simulink library "CTRL_SPECCTRL_FB_STRAT1_REG"  (R2024b)
settings: Solver=VariableStepAuto  StartTime=0.0  StopTime=10.0  RelTol=1e-3
undefined symbols (not defined in the file or in its folder): CTRL_SPECCTRL_FB_STRAT1_REG_DmpLoLim_p100, CTRL_SPECCTRL_FB_STRAT1_REG_DmpUpLim_p100
libraries: slpidlib x4, simulink x4
settings Model: Creator=blatak  LastModifiedBy=blatak

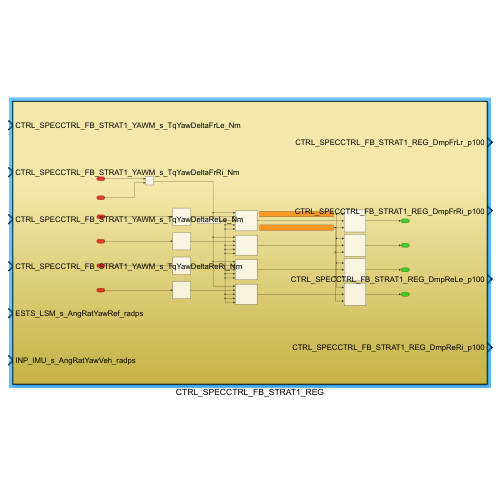
[thumbnail: Simulink's stored preview of the top-level diagram]
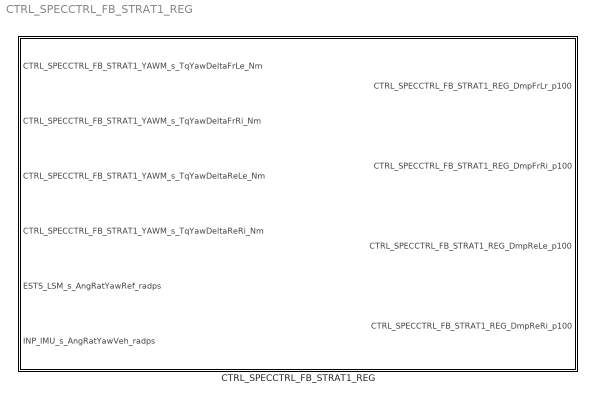
== system CTRL_SPECCTRL_FB_STRAT1_REG ==
  CTRL_SPECCTRL_FB_STRAT1_REG : Subsystem

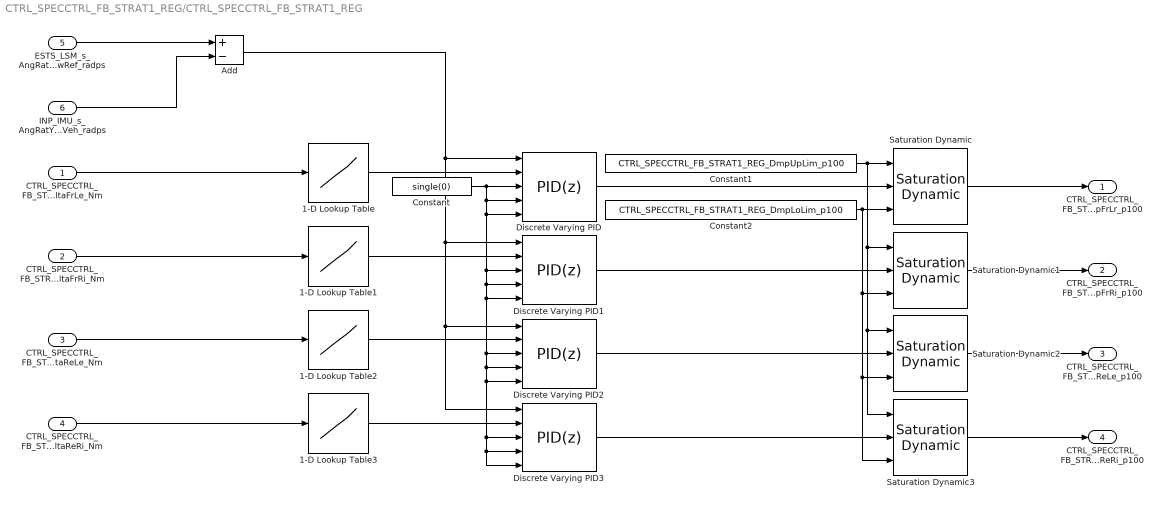
== system CTRL_SPECCTRL_FB_STRAT1_REG/CTRL_SPECCTRL_FB_STRAT1_REG ==
  CTRL_SPECCTRL_FB_STRAT1_YAWM_s_TqYawDeltaFrLe_Nm : Inport
  CTRL_SPECCTRL_FB_STRAT1_YAWM_s_TqYawDeltaFrRi_Nm : Inport  Port=2
  CTRL_SPECCTRL_FB_STRAT1_YAWM_s_TqYawDeltaReLe_Nm : Inport  Port=3
  CTRL_SPECCTRL_FB_STRAT1_YAWM_s_TqYawDeltaReRi_Nm : Inport  Port=4
  ESTS_LSM_s_AngRatYawRef_radps : Inport  Port=5
  INP_IMU_s_AngRatYawVeh_radps : Inport  Port=6
  1-D Lookup Table{,1..3} (4 alike) : Lookup_n-D  NumberOfTableDimensions=1  BreakpointsForDimension1=[-5:5]  Table=tanh([-5:5])  InternalRulePriority=Speed  RndMeth=Simplest
  Add : Sum  Inputs=+-
  Constant : Constant  Value=single(0)
  Constant1 : Constant  Value=CTRL_SPECCTRL_FB_STRAT1_REG_DmpUpLim_p100
  Constant2 : Constant  Value=CTRL_SPECCTRL_FB_STRAT1_REG_DmpLoLim_p100
  Discrete Varying PID{,1..3} (4 alike) : slpidlib/PID Controller  Controller=PID  Form=Parallel  TimeDomain=Discrete-time  UseExternalTs=off  SampleTime=-1  IntegratorMethod=Forward Euler  FilterMethod=Forward Euler  ControllerParametersSource=external  P=1  I=1  UseKiTs=off  D=0  UseExternalDerivativeSource=off  N=100  UseFilter=on  TunerSelectOption=Transfer Function Based (PID Tuner App)  InitialConditionSource=internal  InitialConditionForIntegrator=0  InitialConditionForFilter=0  DifferentiatorICPrevScaledInput=0  ExternalReset=none  TrackingMode=off  Kt=1  LimitOutput=off  SatLimitsSource=internal  UpperSaturationLimit=inf  LowerSaturationLimit=-inf  LinearizeAsGain=on  AntiWindupMode=none  Kb=1  LimitIntegrator=off  UpperIntegratorSaturationLimit=inf  LowerIntegratorSaturationLimit=-inf  POutMin=[]  POutMax=[]  IOutMin=[]  IOutMax=[]  DOutMin=[]  DOutMax=[]  NOutMin=[]  NOutMax=[]  SumOutMin=[]  SumOutMax=[]  SaturationOutMin=[]  SaturationOutMax=[]  PParamMin=[]  PParamMax=[]  IParamMin=[]  IParamMax=[]  DParamMin=[]  DParamMax=[]  NParamMin=[]  NParamMax=[]  KbParamMin=[]  KbParamMax=[]  KtParamMin=[]  KtParamMax=[]  KbOutMin=[]  KbOutMax=[]  KtOutMin=[]  KtOutMax=[]  IntegratorOutMin=[]  IntegratorOutMax=[]  FilterOutMin=[]  FilterOutMax=[]  SumI1OutMin=[]  SumI1OutMax=[]  SumI2OutMin=[]  SumI2OutMax=[]  SumI3OutMin=[]  SumI3OutMax=[]  SumI4OutMin=[]  SumI4OutMax=[]  SumDOutMin=[]  SumDOutMax=[]  DifferentiatorOutMin=[]  DifferentiatorOutMax=[]  FilterDiffOutCoefMin=[]  FilterDiffOutCoefMax=[]  ReciprocalOutMin=[]  ReciprocalOutMax=[]  SumDenOutMin=[]  SumDenOutMax=[]  SumNumOutMin=[]  SumNumOutMax=[]  DivideOutMin=[]  DivideOutMax=[]  UdiffTsProdOutMin=[]  UdiffTsProdOutMax=[]  NTsProdOutMin=[]  NTsProdOutMax=[]  UintegralTsProdOutMin=[]  UintegralTsProdOutMax=[]  UngainTsProdOutMin=[]  UngainTsProdOutMax=[]  ClampingZeroOutDataTypeStr=Inherit: Inherit via back propagation  ClampingZeroOutMin=[]  ClampingZeroOutMax=[]  FilterDenConstantOutDataTypeStr=Inherit: Inherit via back propagation  FilterDenConstantOutMin=[]  FilterDenConstantOutMax=[]  PCopyOutDataTypeStr=Inherit: Inherit via back propagation  PCopyOutMin=[]  PCopyOutMax=[]  NCopyOutDataTypeStr=Inherit: Inherit via back propagation  NCopyOutMin=[]  NCopyOutMax=[]  IntegratorContinuousStateAttributes=''  IntegratorStateMustResolveToSignalObject=off  IntegratorRTWStateStorageClass=Auto  FilterContinuousStateAttributes=''  FilterStateMustResolveToSignalObject=off  FilterRTWStateStorageClass=Auto  ParallelPVariant=ExternalParameters  IdealPVariant=Disabled  IVariant=ExternalParameters  DVariant=ExternalParameters  IntegratorVariant=Discrete  SatVariant=Disabled  AWVariant=Passthrough  PCopyVariant=Disabled  TRVariant=Disabled  FdbkBlocksVariant=Forward  IdealPFdbkVariant=Disabled  SatFdbkVariant=Disabled  DerivativeFilterVariant=ForwardEulerFilter  NVariant=ExternalParameters  NCopyVariant=Disabled  FilterICVariant=InternalICsFilter  IntegratorICVariant=InternalICs  ExternalResetVariant=Disabled  TRSumVariant=Passthrough  SumFdbkVariant=Disabled  SumVariant=Sum_PID  TsampFilterVariant=InternalTs  TsampNgainVariant=Passthrough  TsampIntegralVariant=Disabled_SignalSpec  ExternalSaturationOutDataTypeStr=Inherit: Same as second input  DerivativeSourceVariant=ErrorSignal  PreIntVariant=InternalPreInt
      settings: LibrarySourceBlock=cstblocks/Linear Parameter Varying/Discrete Varying PID
  Saturation Dynamic{,1..3} (4 alike) : simulink/Discontinuities/Saturation Dynamic  OutMin=[]  OutMax=[]  OutDataTypeStr=Inherit: Same as second input  OutDataType=fixdt(1, 16)  OutScaling=2^-10  DoSatur=off
  CTRL_SPECCTRL_FB_STRAT1_REG_DmpFrLr_p100 : Outport
  CTRL_SPECCTRL_FB_STRAT1_REG_DmpFrRi_p100 : Outport  Port=2
  CTRL_SPECCTRL_FB_STRAT1_REG_DmpReLe_p100 : Outport  Port=3
  CTRL_SPECCTRL_FB_STRAT1_REG_DmpReRi_p100 : Outport  Port=4
  wires:
  Constant2/1 -> Saturation Dynamic3/3, Saturation Dynamic2/3, Saturation Dynamic1/3, Saturation Dynamic/3
  ESTS_LSM_s_AngRatYawRef_radps/1 -> Add/1
  Saturation Dynamic3/1 -> CTRL_SPECCTRL_FB_STRAT1_REG_DmpReRi_p100/1
  Constant1/1 -> Saturation Dynamic3/1, Saturation Dynamic2/1, Saturation Dynamic1/1, Saturation Dynamic/1
  CTRL_SPECCTRL_FB_STRAT1_YAWM_s_TqYawDeltaFrRi_Nm/1 -> 1-D Lookup Table1/1
  Add/1 -> Discrete Varying PID3/1, Discrete Varying PID2/1, Discrete Varying PID1/1, Discrete Varying PID/1
  1-D Lookup Table3/1 -> Discrete Varying PID3/2
  Constant/1 -> Discrete Varying PID/4, Discrete Varying PID/5, Discrete Varying PID1/4, Discrete Varying PID1/5, Discrete Varying PID2/4, Discrete Varying PID2/5, Discrete Varying PID3/5, Discrete Varying PID3/4, Discrete Varying PID3/3, Discrete Varying PID2/3, Discrete Varying PID1/3, Discrete Varying PID/3
  Saturation Dynamic/1 -> CTRL_SPECCTRL_FB_STRAT1_REG_DmpFrLr_p100/1
  1-D Lookup Table1/1 -> Discrete Varying PID1/2
  Discrete Varying PID2/1 -> Saturation Dynamic2/2
  1-D Lookup Table/1 -> Discrete Varying PID/2
  CTRL_SPECCTRL_FB_STRAT1_YAWM_s_TqYawDeltaFrLe_Nm/1 -> 1-D Lookup Table/1
  INP_IMU_s_AngRatYawVeh_radps/1 -> Add/2
  Saturation Dynamic1/1 -> CTRL_SPECCTRL_FB_STRAT1_REG_DmpFrRi_p100/1
  Discrete Varying PID1/1 -> Saturation Dynamic1/2
  1-D Lookup Table2/1 -> Discrete Varying PID2/2
  Saturation Dynamic2/1 -> CTRL_SPECCTRL_FB_STRAT1_REG_DmpReLe_p100/1
  CTRL_SPECCTRL_FB_STRAT1_YAWM_s_TqYawDeltaReLe_Nm/1 -> 1-D Lookup Table2/1
  CTRL_SPECCTRL_FB_STRAT1_YAWM_s_TqYawDeltaReRi_Nm/1 -> 1-D Lookup Table3/1
  Discrete Varying PID3/1 -> Saturation Dynamic3/2
  Discrete Varying PID/1 -> Saturation Dynamic/2
